simulink model "model_13"  (R2022b)
settings: Solver=VariableStepAuto  StartTime=0.0  StopTime=2000  FixedStep=1e-3  RelTol=1e-3  EnableMultiTasking=on
StopFcn:
  | ee_addSimlogTimeStamp(bdroot)
libraries: fl_lib x74, nesl_utility x53, ee_lib x22, spsRMSLib x22, eePowerMeasurement x11
(part 1 of 2)
CloseFcn:
  | try,close(h1_ee_voltreg_linear_feedback),end
  | clear h1_ee_voltreg_linear_feedback
  | try,close(h2_ee_voltreg_linear_feedback),end
  | 
  | clear simlog_ee_voltreg_linear_feedback
  | clear logsout_ee_voltreg_linear_feedback
  | clear tout
Description:
  | Linear Voltage Regulator with Feedback
settings Model: Creator=The MathWorks, Inc.  LastModifiedBy=aykut
settings SolverCC: ZeroCrossAlgorithm=Adaptive  AlgebraicLoopSolver=TrustRegion
settings DataIOCC: MaxDataPoints=15000  SaveFormat=Array  ReturnWorkspaceOutputs=off  SignalLoggingName=logsout_ee_voltreg_linear_feedback
settings OptimizationCC: ExpressionDepthLimit=2147483647  InitFltsAndDblsToZero=on  LifeSpan=inf
settings DebuggingCC: SaveWithParameterizedLinksMsg=none  UnderspecifiedInitializationDetection=Classic  MergeDetectMultiDrivingBlocksExec=none  IgnoredZcDiagnostic=none  FcnCallInpInsideContextMsg=warning  UnconnectedInputMsg=warning  UnconnectedOutputMsg=warning  UnconnectedLineMsg=warning  StateNameClashWarn=warning  SFUnexpectedBacktrackingDiag=warning  SFNoUnconditionalDefaultTransitionDiag=warning  SFExecutionAtInitializationDiag=none  SFMachineParentedDataDiag=warning  ArithmeticOperatorsInVariantConditions=warning
settings HardwareCC: ProdBitPerPointer=32  ProdBitPerSizeT=32  ProdBitPerPtrDiffT=32  ProdLargestAtomicFloat=None  ProdIntDivRoundTo=Undefined  ProdEndianess=Unspecified  ProdWordSize=32  ProdHWDeviceType=32-bit Generic
settings ModelReferenceCC: EnableRefExpFcnMdlSchedulingChecks=on  PropagateSignalLabelsOutOfModel=off
settings SFSimCC: SimUseLocalCustomCode=off  CustomCodeUndefinedFunction=UseInterfaceOnly
settings RTWCC: RTWUseLocalCustomCode=off  DLArmComputeVersion=19.05
settings CodeAppCC: StateflowObjectComments=on
settings GRTTargetCC: TargetFcnLib=ansi_tfl_tmw.mat  TargetLangStandard=C89/C90 (ANSI)  CombineOutputUpdateFcns=off  GRTInterface=on
settings ConfigComp: CovMetricSettings=dw  CovSaveCumulativeToWorkspaceVar=on  CovSaveSingleToWorkspaceVar=on  CovExternalEMLEnable=off  CovSFcnEnable=off
settings SimscapeCC: SimscapeLogType=all  SimscapeLogSimulationStatistics=on  SimscapeLogName=simlog_ee_voltreg_linear_feedback  SimscapeLogDataHistory=15000

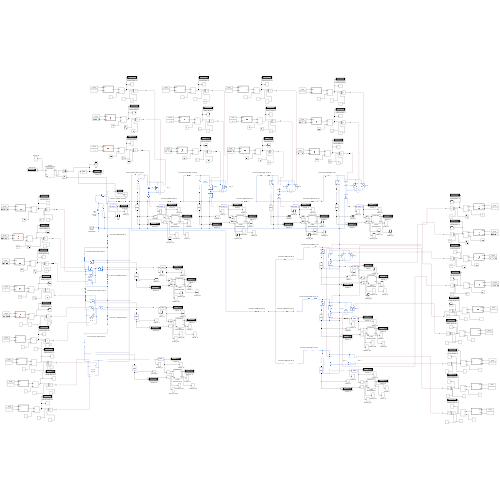
[thumbnail: Simulink's stored preview of the top-level diagram]
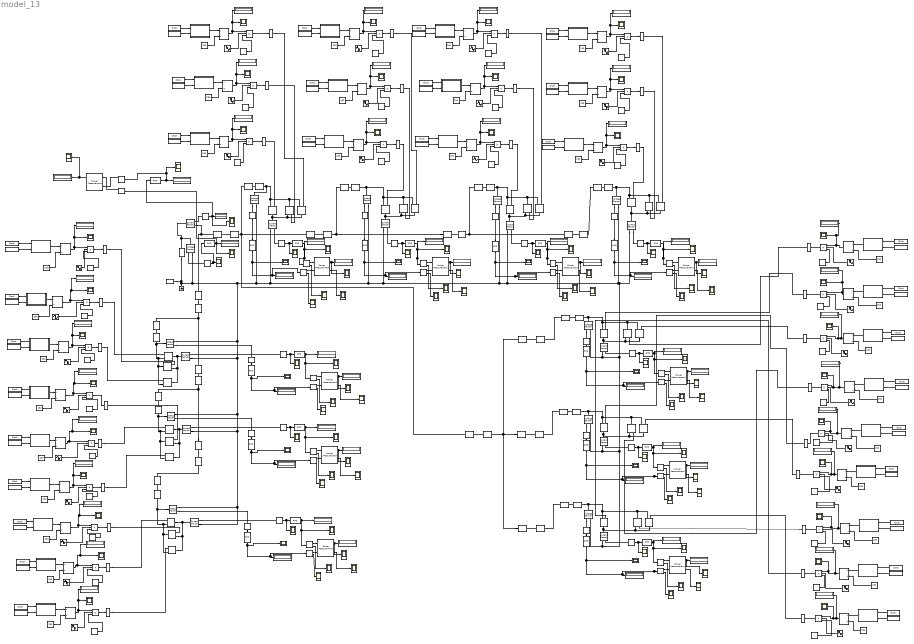
== system model_13 ==
  -Line Pair 10 (AMKA 35 52 m) : fl_lib/Electrical/Electrical Elements/Resistor  R=0.045136 Ohm  i_specify=off  i_priority=High  i=0 A  i_nominal_specify=off  i_nominal_unit=A  i_nominal_value=1  v_specify=off  v_priority=High  v=0 V  v_nominal_specify=off  v_nominal_unit=V  v_nominal_value=1
  -Line Pair 11 (AMKA 25 58 m) : fl_lib/Electrical/Electrical Elements/Resistor  R=0.0696 Ohm  i_specify=off  i_priority=High  i=0 A  i_nominal_specify=off  i_nominal_unit=A  i_nominal_value=1  v_specify=off  v_priority=High  v=0 V  v_nominal_specify=off  v_nominal_unit=V  v_nominal_value=1
  -Line Pair 9 (AMKA 35 85 m) : fl_lib/Electrical/Electrical Elements/Resistor  R=0.07378 Ohm  i_specify=off  i_priority=High  i=0 A  i_nominal_specify=off  i_nominal_unit=A  i_nominal_value=1  v_specify=off  v_priority=High  v=0 V  v_nominal_specify=off  v_nominal_unit=V  v_nominal_value=1
  -Line Pair House 2(MC 10 48 m) : fl_lib/Electrical/Electrical Elements/Resistor  R=0.08784 Ohm  i_specify=off  i_priority=High  i=0 A  i_nominal_specify=off  i_nominal_unit=A  i_nominal_value=1  v_specify=off  v_priority=High  v=0 V  v_nominal_specify=off  v_nominal_unit=V  v_nominal_value=1
  -Line Pair House 3(MC 10 34 m) : fl_lib/Electrical/Electrical Elements/Resistor  R=0.06222 Ohm  i_specify=off  i_priority=High  i=0 A  i_nominal_specify=off  i_nominal_unit=A  i_nominal_value=1  v_specify=off  v_priority=High  v=0 V  v_nominal_specify=off  v_nominal_unit=V  v_nominal_value=1
  -Line Pair House 4(MC6  4 m) : fl_lib/Electrical/Electrical Elements/Resistor  R=0.01232 Ohm  i_specify=off  i_priority=High  i=0 A  i_nominal_specify=off  i_nominal_unit=A  i_nominal_value=1  v_specify=off  v_priority=High  v=0 V  v_nominal_specify=off  v_nominal_unit=V  v_nominal_value=1
  -Line Pair House 5(MC 6 11 m) : fl_lib/Electrical/Electrical Elements/Resistor  R=0.03388 Ohm  i_specify=off  i_priority=High  i=0 A  i_nominal_specify=off  i_nominal_unit=A  i_nominal_value=1  v_specify=off  v_priority=High  v=0 V  v_nominal_specify=off  v_nominal_unit=V  v_nominal_value=1
  -Line Pair House 6(MC 10 12 m) : fl_lib/Electrical/Electrical Elements/Resistor  R=0.02196 Ohm  i_specify=off  i_priority=High  i=0 A  i_nominal_specify=off  i_nominal_unit=A  i_nominal_value=1  v_specify=off  v_priority=High  v=0 V  v_nominal_specify=off  v_nominal_unit=V  v_nominal_value=1
  Complex to Real-Imag{1..22} (22 alike) : ComplexToRealImag
  Constant{1..30} (30 alike) : Constant  Value=230
  Constant{31..60} (30 alike) : Constant  Value=sqrt(2)
  Controlled Current Source{,1..9} (10 alike) : fl_lib/Electrical/Electrical Sources/Controlled Current Source
  Current Sensor{,1..10} (11 alike) : fl_lib/Electrical/Electrical Sensors/Current Sensor
  Digital Clock{1..30} (30 alike) : DigitalClock
  Divide{1..30} (30 alike) : Product  Inputs=*/
  ERef : fl_lib/Electrical/Electrical Elements/Electrical Reference
  EV_{1..10} (10 alike) : fl_lib/Electrical/Electrical Sources/Controlled Current Source
  From Workspace : FromWorkspace  VariableName=house1_load_array  OutDataTypeStr=double  Interpolate=off  OutputAfterFinalValue=Holding final value
  From Workspace1 : FromWorkspace  VariableName=house1_pv_array  OutDataTypeStr=double  Interpolate=off  OutputAfterFinalValue=Holding final value
  From Workspace10 : FromWorkspace  VariableName=house9_load_array  OutDataTypeStr=double  Interpolate=off  OutputAfterFinalValue=Holding final value
  From Workspace11 : FromWorkspace  VariableName=house9_pv_array  OutDataTypeStr=double  Interpolate=off  OutputAfterFinalValue=Holding final value
  From Workspace12 : FromWorkspace  VariableName=house10_load_array  OutDataTypeStr=double  Interpolate=off  OutputAfterFinalValue=Holding final value
  From Workspace13 : FromWorkspace  VariableName=house10_pv_array  OutDataTypeStr=double  Interpolate=off  OutputAfterFinalValue=Holding final value
  From Workspace14 : FromWorkspace  VariableName=house5_load_array  OutDataTypeStr=double  Interpolate=off  OutputAfterFinalValue=Holding final value
  From Workspace15 : FromWorkspace  VariableName=house5_pv_array  OutDataTypeStr=double  Interpolate=off  OutputAfterFinalValue=Holding final value
  From Workspace16 : FromWorkspace  VariableName=house6_load_array  OutDataTypeStr=double  Interpolate=off  OutputAfterFinalValue=Holding final value
  From Workspace17 : FromWorkspace  VariableName=house6_pv_array  OutDataTypeStr=double  Interpolate=off  OutputAfterFinalValue=Holding final value
  From Workspace18 : FromWorkspace  VariableName=house7_load_array  OutDataTypeStr=double  Interpolate=off  OutputAfterFinalValue=Holding final value
  From Workspace19 : FromWorkspace  VariableName=house7_pv_array  OutDataTypeStr=double  Interpolate=off  OutputAfterFinalValue=Holding final value
  From Workspace2 : FromWorkspace  VariableName=house2_load_array  OutDataTypeStr=double  Interpolate=off  OutputAfterFinalValue=Holding final value
  From Workspace20 : FromWorkspace  VariableName=house1_ev_array  OutDataTypeStr=double  Interpolate=off  OutputAfterFinalValue=Holding final value
  From Workspace21 : FromWorkspace  VariableName=house2_ev_array  OutDataTypeStr=double  Interpolate=off  OutputAfterFinalValue=Holding final value
  From Workspace22 : FromWorkspace  VariableName=house3_ev_array  OutDataTypeStr=double  Interpolate=off  OutputAfterFinalValue=Holding final value
  From Workspace23 : FromWorkspace  VariableName=house4_ev_array  OutDataTypeStr=double  Interpolate=off  OutputAfterFinalValue=Holding final value
  From Workspace24 : FromWorkspace  VariableName=house5_ev_array  OutDataTypeStr=double  Interpolate=off  OutputAfterFinalValue=Holding final value
  From Workspace25 : FromWorkspace  VariableName=house6_ev_array  OutDataTypeStr=double  Interpolate=off  OutputAfterFinalValue=Holding final value
  From Workspace26 : FromWorkspace  VariableName=house7_ev_array  OutDataTypeStr=double  Interpolate=off  OutputAfterFinalValue=Holding final value
  From Workspace27 : FromWorkspace  VariableName=house8_ev_array  OutDataTypeStr=double  Interpolate=off  OutputAfterFinalValue=Holding final value
  From Workspace28 : FromWorkspace  VariableName=house9_ev_array  OutDataTypeStr=double  Interpolate=off  OutputAfterFinalValue=Holding final value
  From Workspace29 : FromWorkspace  VariableName=house10_ev_array  OutDataTypeStr=double  Interpolate=off  OutputAfterFinalValue=Holding final value
  From Workspace3 : FromWorkspace  VariableName=house2_pv_array  OutDataTypeStr=double  Interpolate=off  OutputAfterFinalValue=Holding final value
  From Workspace4 : FromWorkspace  VariableName=house3_load_array  OutDataTypeStr=double  Interpolate=off  OutputAfterFinalValue=Holding final value
  From Workspace5 : FromWorkspace  VariableName=house3_pv_array  OutDataTypeStr=double  Interpolate=off  OutputAfterFinalValue=Holding final value
  From Workspace6 : FromWorkspace  VariableName=house4_load_array  OutDataTypeStr=double  Interpolate=off  OutputAfterFinalValue=Holding final value
  From Workspace7 : FromWorkspace  VariableName=house4_pv_array  OutDataTypeStr=double  Interpolate=off  OutputAfterFinalValue=Holding final value
  From Workspace8 : FromWorkspace  VariableName=house8_load_array  OutDataTypeStr=double  Interpolate=off  OutputAfterFinalValue=Holding final value
  From Workspace9 : FromWorkspace  VariableName=house8_pv_array  OutDataTypeStr=double  Interpolate=off  OutputAfterFinalValue=Holding final value
  Ih10rms_d : Display
  Ih10rms_s1 : Scope
  Ih10rms_s2 : Scope
  Ih1rms_d{,1..3} (4 alike) : Display
  Ih1rms_s1 : Scope
  Ih1rms_s2 : Scope
  Ih1rms_s3 : Scope
  Ih2rms_d : Display
  Ih2rms_s1 : Scope
  Ih2rms_s2 : Scope
  Ih3rms_d : Display
  Ih3rms_s1 : Scope
  Ih3rms_s2 : Scope
  Ih4rms_d : Display
  Ih4rms_s1 : Scope
  Ih4rms_s2 : Scope
  Ih5rms_d : Display
  Ih5rms_s1 : Scope
  Ih5rms_s2 : Scope
  Ih6rms_d : Display
  Ih6rms_s1 : Scope
  Ih6rms_s2 : Scope
  Ih7rms_d : Display
  Ih7rms_s1 : Scope
  Ih7rms_s2 : Scope
  Ih8rms_d : Display
  Ih8rms_s1 : Scope
  Ih8rms_s2 : Scope
  Ih9rms_d : Display
  Ih9rms_s1 : Scope
  Ih9rms_s2 : Scope
  Inductor : ee_lib/Passive/Inductor  l=2.947770700636943e-5 H  enable_L_tol=0  L_tol=20  tol_distribution=1  nSigma=4  r=0 Ohm  g=0 1/Ohm  enable_operating_limits=0  operating_limit_action=2  max_working_current=1 A  power_rating=1 W  enable_faults=0  fault_action=1  lambdaPercent=50  k_faulted=0.9999  turnsShort=0  openCct=0  groundShort=0  groundShortG=0 1/Ohm  tau_fault=1e-3 s  enable_temporal_fault=0  t_fault=1 s  enable_behavioral_fault=0  max_permissible_voltage=100 V  n_fail_on_voltage=1  max_permissible_current=1 A  t_fail_on_current=1 s  i_L_specify=off  i_L_priority=High  i_L=0 A  i_L_nominal_specify=off  i_L_nominal_unit=A  i_L_nominal_value=1
  Inductor1 : ee_lib/Passive/Inductor  l=1.064968152866242e-5 H  enable_L_tol=0  L_tol=20  tol_distribution=1  nSigma=4  r=0 Ohm  g=0 1/Ohm  enable_operating_limits=0  operating_limit_action=2  max_working_current=1 A  power_rating=1 W  enable_faults=0  fault_action=1  lambdaPercent=50  k_faulted=0.9999  turnsShort=0  openCct=0  groundShort=0  groundShortG=0 1/Ohm  tau_fault=1e-3 s  enable_temporal_fault=0  t_fault=1 s  enable_behavioral_fault=0  max_permissible_voltage=100 V  n_fail_on_voltage=1  max_permissible_current=1 A  t_fail_on_current=1 s  i_L_specify=off  i_L_priority=High  i_L=0 A  i_L_nominal_specify=off  i_L_nominal_unit=A  i_L_nominal_value=1
  Inductor10 : ee_lib/Passive/Inductor  l=1.547770700636943e-5 H  enable_L_tol=0  L_tol=20  tol_distribution=1  nSigma=4  r=0 Ohm  g=0 1/Ohm  enable_operating_limits=0  operating_limit_action=2  max_working_current=1 A  power_rating=1 W  enable_faults=0  fault_action=1  lambdaPercent=50  k_faulted=0.9999  turnsShort=0  openCct=0  groundShort=0  groundShortG=0 1/Ohm  tau_fault=1e-3 s  enable_temporal_fault=0  t_fault=1 s  enable_behavioral_fault=0  max_permissible_voltage=100 V  n_fail_on_voltage=1  max_permissible_current=1 A  t_fail_on_current=1 s  i_L_specify=off  i_L_priority=High  i_L=0 A  i_L_nominal_specify=off  i_L_nominal_unit=A  i_L_nominal_value=1
  Inductor11 : ee_lib/Passive/Inductor  l=4.537579617834395e-5 H  enable_L_tol=0  L_tol=20  tol_distribution=1  nSigma=4  r=0 Ohm  g=0 1/Ohm  enable_operating_limits=0  operating_limit_action=2  max_working_current=1 A  power_rating=1 W  enable_faults=0  fault_action=1  lambdaPercent=50  k_faulted=0.9999  turnsShort=0  openCct=0  groundShort=0  groundShortG=0 1/Ohm  tau_fault=1e-3 s  enable_temporal_fault=0  t_fault=1 s  enable_behavioral_fault=0  max_permissible_voltage=100 V  n_fail_on_voltage=1  max_permissible_current=1 A  t_fail_on_current=1 s  i_L_specify=off  i_L_priority=High  i_L=0 A  i_L_nominal_specify=off  i_L_nominal_unit=A  i_L_nominal_value=1
  Inductor12 : ee_lib/Passive/Inductor  l=1.092993630573248e-5 H  enable_L_tol=0  L_tol=20  tol_distribution=1  nSigma=4  r=0 Ohm  g=0 1/Ohm  enable_operating_limits=0  operating_limit_action=2  max_working_current=1 A  power_rating=1 W  enable_faults=0  fault_action=1  lambdaPercent=50  k_faulted=0.9999  turnsShort=0  openCct=0  groundShort=0  groundShortG=0 1/Ohm  tau_fault=1e-3 s  enable_temporal_fault=0  t_fault=1 s  enable_behavioral_fault=0  max_permissible_voltage=100 V  n_fail_on_voltage=1  max_permissible_current=1 A  t_fail_on_current=1 s  i_L_specify=off  i_L_priority=High  i_L=0 A  i_L_nominal_specify=off  i_L_nominal_unit=A  i_L_nominal_value=1
  Inductor13 : ee_lib/Passive/Inductor  l=3.152866242038217e-6 H  enable_L_tol=0  L_tol=20  tol_distribution=1  nSigma=4  r=0 Ohm  g=0 1/Ohm  enable_operating_limits=0  operating_limit_action=2  max_working_current=1 A  power_rating=1 W  enable_faults=0  fault_action=1  lambdaPercent=50  k_faulted=0.9999  turnsShort=0  openCct=0  groundShort=0  groundShortG=0 1/Ohm  tau_fault=1e-3 s  enable_temporal_fault=0  t_fault=1 s  enable_behavioral_fault=0  max_permissible_voltage=100 V  n_fail_on_voltage=1  max_permissible_current=1 A  t_fail_on_current=1 s  i_L_specify=off  i_L_priority=High  i_L=0 A  i_L_nominal_specify=off  i_L_nominal_unit=A  i_L_nominal_value=1
  Inductor14 : ee_lib/Passive/Inductor  l=3.363057324840764e-6 H  enable_L_tol=0  L_tol=20  tol_distribution=1  nSigma=4  r=0 Ohm  g=0 1/Ohm  enable_operating_limits=0  operating_limit_action=2  max_working_current=1 A  power_rating=1 W  enable_faults=0  fault_action=1  lambdaPercent=50  k_faulted=0.9999  turnsShort=0  openCct=0  groundShort=0  groundShortG=0 1/Ohm  tau_fault=1e-3 s  enable_temporal_fault=0  t_fault=1 s  enable_behavioral_fault=0  max_permissible_voltage=100 V  n_fail_on_voltage=1  max_permissible_current=1 A  t_fail_on_current=1 s  i_L_specify=off  i_L_priority=High  i_L=0 A  i_L_nominal_specify=off  i_L_nominal_unit=A  i_L_nominal_value=1
  Inductor15 : ee_lib/Passive/Inductor  l=1.064968152866242e-5 H  enable_L_tol=0  L_tol=20  tol_distribution=1  nSigma=4  r=0 Ohm  g=0 1/Ohm  enable_operating_limits=0  operating_limit_action=2  max_working_current=1 A  power_rating=1 W  enable_faults=0  fault_action=1  lambdaPercent=50  k_faulted=0.9999  turnsShort=0  openCct=0  groundShort=0  groundShortG=0 1/Ohm  tau_fault=1e-3 s  enable_temporal_fault=0  t_fault=1 s  enable_behavioral_fault=0  max_permissible_voltage=100 V  n_fail_on_voltage=1  max_permissible_current=1 A  t_fail_on_current=1 s  i_L_specify=off  i_L_priority=High  i_L=0 A  i_L_nominal_specify=off  i_L_nominal_unit=A  i_L_nominal_value=1
  Inductor16 : ee_lib/Passive/Inductor  l=8.127388535031847e-6 H  enable_L_tol=0  L_tol=20  tol_distribution=1  nSigma=4  r=0 Ohm  g=0 1/Ohm  enable_operating_limits=0  operating_limit_action=2  max_working_current=1 A  power_rating=1 W  enable_faults=0  fault_action=1  lambdaPercent=50  k_faulted=0.9999  turnsShort=0  openCct=0  groundShort=0  groundShortG=0 1/Ohm  tau_fault=1e-3 s  enable_temporal_fault=0  t_fault=1 s  enable_behavioral_fault=0  max_permissible_voltage=100 V  n_fail_on_voltage=1  max_permissible_current=1 A  t_fail_on_current=1 s  i_L_specify=off  i_L_priority=High  i_L=0 A  i_L_nominal_specify=off  i_L_nominal_unit=A  i_L_nominal_value=1
  Inductor17 : ee_lib/Passive/Inductor  l=1.722292993630573e-5 H  enable_L_tol=0  L_tol=20  tol_distribution=1  nSigma=4  r=0 Ohm  g=0 1/Ohm  enable_operating_limits=0  operating_limit_action=2  max_working_current=1 A  power_rating=1 W  enable_faults=0  fault_action=1  lambdaPercent=50  k_faulted=0.9999  turnsShort=0  openCct=0  groundShort=0  groundShortG=0 1/Ohm  tau_fault=1e-3 s  enable_temporal_fault=0  t_fault=1 s  enable_behavioral_fault=0  max_permissible_voltage=100 V  n_fail_on_voltage=1  max_permissible_current=1 A  t_fail_on_current=1 s  i_L_specify=off  i_L_priority=High  i_L=0 A  i_L_nominal_specify=off  i_L_nominal_unit=A  i_L_nominal_value=1
  Inductor18 : ee_lib/Passive/Inductor  l=9.808917197452229e-6 H  enable_L_tol=0  L_tol=20  tol_distribution=1  nSigma=4  r=0 Ohm  g=0 1/Ohm  enable_operating_limits=0  operating_limit_action=2  max_working_current=1 A  power_rating=1 W  enable_faults=0  fault_action=1  lambdaPercent=50  k_faulted=0.9999  turnsShort=0  openCct=0  groundShort=0  groundShortG=0 1/Ohm  tau_fault=1e-3 s  enable_temporal_fault=0  t_fault=1 s  enable_behavioral_fault=0  max_permissible_voltage=100 V  n_fail_on_voltage=1  max_permissible_current=1 A  t_fail_on_current=1 s  i_L_specify=off  i_L_priority=High  i_L=0 A  i_L_nominal_specify=off  i_L_nominal_unit=A  i_L_nominal_value=1
  Inductor19 : ee_lib/Passive/Inductor  l=1.95796178343949e-5 H  enable_L_tol=0  L_tol=20  tol_distribution=1  nSigma=4  r=0 Ohm  g=0 1/Ohm  enable_operating_limits=0  operating_limit_action=2  max_working_current=1 A  power_rating=1 W  enable_faults=0  fault_action=1  lambdaPercent=50  k_faulted=0.9999  turnsShort=0  openCct=0  groundShort=0  groundShortG=0 1/Ohm  tau_fault=1e-3 s  enable_temporal_fault=0  t_fault=1 s  enable_behavioral_fault=0  max_permissible_voltage=100 V  n_fail_on_voltage=1  max_permissible_current=1 A  t_fail_on_current=1 s  i_L_specify=off  i_L_priority=High  i_L=0 A  i_L_nominal_specify=off  i_L_nominal_unit=A  i_L_nominal_value=1
  Inductor2 : ee_lib/Passive/Inductor  l=1.987261146496815e-5 H  enable_L_tol=0  L_tol=20  tol_distribution=1  nSigma=4  r=0 Ohm  g=0 1/Ohm  enable_operating_limits=0  operating_limit_action=2  max_working_current=1 A  power_rating=1 W  enable_faults=0  fault_action=1  lambdaPercent=50  k_faulted=0.9999  turnsShort=0  openCct=0  groundShort=0  groundShortG=0 1/Ohm  tau_fault=1e-3 s  enable_temporal_fault=0  t_fault=1 s  enable_behavioral_fault=0  max_permissible_voltage=100 V  n_fail_on_voltage=1  max_permissible_current=1 A  t_fail_on_current=1 s  i_L_specify=off  i_L_priority=High  i_L=0 A  i_L_nominal_specify=off  i_L_nominal_unit=A  i_L_nominal_value=1
  Inductor20 : ee_lib/Passive/Inductor  l=1.146496815286624e-5 H  enable_L_tol=0  L_tol=20  tol_distribution=1  nSigma=4  r=0 Ohm  g=0 1/Ohm  enable_operating_limits=0  operating_limit_action=2  max_working_current=1 A  power_rating=1 W  enable_faults=0  fault_action=1  lambdaPercent=50  k_faulted=0.9999  turnsShort=0  openCct=0  groundShort=0  groundShortG=0 1/Ohm  tau_fault=1e-3 s  enable_temporal_fault=0  t_fault=1 s  enable_behavioral_fault=0  max_permissible_voltage=100 V  n_fail_on_voltage=1  max_permissible_current=1 A  t_fail_on_current=1 s  i_L_specify=off  i_L_priority=High  i_L=0 A  i_L_nominal_specify=off  i_L_nominal_unit=A  i_L_nominal_value=1
  Inductor3 : ee_lib/Passive/Inductor  l=3.146496815286624e-5 H  enable_L_tol=0  L_tol=20  tol_distribution=1  nSigma=4  r=0 Ohm  g=0 1/Ohm  enable_operating_limits=0  operating_limit_action=2  max_working_current=1 A  power_rating=1 W  enable_faults=0  fault_action=1  lambdaPercent=50  k_faulted=0.9999  turnsShort=0  openCct=0  groundShort=0  groundShortG=0 1/Ohm  tau_fault=1e-3 s  enable_temporal_fault=0  t_fault=1 s  enable_behavioral_fault=0  max_permissible_voltage=100 V  n_fail_on_voltage=1  max_permissible_current=1 A  t_fail_on_current=1 s  i_L_specify=off  i_L_priority=High  i_L=0 A  i_L_nominal_specify=off  i_L_nominal_unit=A  i_L_nominal_value=1
  Inductor4 : ee_lib/Passive/Inductor  l=1.600254777070064e-4 H  enable_L_tol=0  L_tol=20  tol_distribution=1  nSigma=4  r=0 Ohm  g=0 1/Ohm  enable_operating_limits=0  operating_limit_action=2  max_working_current=1 A  power_rating=1 W  enable_faults=0  fault_action=1  lambdaPercent=50  k_faulted=0.9999  turnsShort=0  openCct=0  groundShort=0  groundShortG=0 1/Ohm  tau_fault=1e-3 s  enable_temporal_fault=0  t_fault=1 s  enable_behavioral_fault=0  max_permissible_voltage=100 V  n_fail_on_voltage=1  max_permissible_current=1 A  t_fail_on_current=1 s  i_L_specify=off  i_L_priority=High  i_L=0 A  i_L_nominal_specify=off  i_L_nominal_unit=A  i_L_nominal_value=1
  Inductor5 : ee_lib/Passive/Inductor  l=1.345222929936306e-5 H  enable_L_tol=0  L_tol=20  tol_distribution=1  nSigma=4  r=0 Ohm  g=0 1/Ohm  enable_operating_limits=0  operating_limit_action=2  max_working_current=1 A  power_rating=1 W  enable_faults=0  fault_action=1  lambdaPercent=50  k_faulted=0.9999  turnsShort=0  openCct=0  groundShort=0  groundShortG=0 1/Ohm  tau_fault=1e-3 s  enable_temporal_fault=0  t_fault=1 s  enable_behavioral_fault=0  max_permissible_voltage=100 V  n_fail_on_voltage=1  max_permissible_current=1 A  t_fail_on_current=1 s  i_L_specify=off  i_L_priority=High  i_L=0 A  i_L_nominal_specify=off  i_L_nominal_unit=A  i_L_nominal_value=1
  Inductor6 : ee_lib/Passive/Inductor  l=9.528662420382166e-6 H  enable_L_tol=0  L_tol=20  tol_distribution=1  nSigma=4  r=0 Ohm  g=0 1/Ohm  enable_operating_limits=0  operating_limit_action=2  max_working_current=1 A  power_rating=1 W  enable_faults=0  fault_action=1  lambdaPercent=50  k_faulted=0.9999  turnsShort=0  openCct=0  groundShort=0  groundShortG=0 1/Ohm  tau_fault=1e-3 s  enable_temporal_fault=0  t_fault=1 s  enable_behavioral_fault=0  max_permissible_voltage=100 V  n_fail_on_voltage=1  max_permissible_current=1 A  t_fail_on_current=1 s  i_L_specify=off  i_L_priority=High  i_L=0 A  i_L_nominal_specify=off  i_L_nominal_unit=A  i_L_nominal_value=1
  Inductor7 : ee_lib/Passive/Inductor  l=1.146496815286624e-6 H  enable_L_tol=0  L_tol=20  tol_distribution=1  nSigma=4  r=0 Ohm  g=0 1/Ohm  enable_operating_limits=0  operating_limit_action=2  max_working_current=1 A  power_rating=1 W  enable_faults=0  fault_action=1  lambdaPercent=50  k_faulted=0.9999  turnsShort=0  openCct=0  groundShort=0  groundShortG=0 1/Ohm  tau_fault=1e-3 s  enable_temporal_fault=0  t_fault=1 s  enable_behavioral_fault=0  max_permissible_voltage=100 V  n_fail_on_voltage=1  max_permissible_current=1 A  t_fail_on_current=1 s  i_L_specify=off  i_L_priority=High  i_L=0 A  i_L_nominal_specify=off  i_L_nominal_unit=A  i_L_nominal_value=1
  Inductor8 : ee_lib/Passive/Inductor  l=0.0000273407643312 H  enable_L_tol=0  L_tol=20  tol_distribution=1  nSigma=4  r=0 Ohm  g=0 1/Ohm  enable_operating_limits=0  operating_limit_action=2  max_working_current=1 A  power_rating=1 W  enable_faults=0  fault_action=1  lambdaPercent=50  k_faulted=0.9999  turnsShort=0  openCct=0  groundShort=0  groundShortG=0 1/Ohm  tau_fault=1e-3 s  enable_temporal_fault=0  t_fault=1 s  enable_behavioral_fault=0  max_permissible_voltage=100 V  n_fail_on_voltage=1  max_permissible_current=1 A  t_fail_on_current=1 s  i_L_specify=off  i_L_priority=High  i_L=0 A  i_L_nominal_specify=off  i_L_nominal_unit=A  i_L_nominal_value=1
  Inductor9 : ee_lib/Passive/Inductor  l=8.214012738853503e-5 H  enable_L_tol=0  L_tol=20  tol_distribution=1  nSigma=4  r=0 Ohm  g=0 1/Ohm  enable_operating_limits=0  operating_limit_action=2  max_working_current=1 A  power_rating=1 W  enable_faults=0  fault_action=1  lambdaPercent=50  k_faulted=0.9999  turnsShort=0  openCct=0  groundShort=0  groundShortG=0 1/Ohm  tau_fault=1e-3 s  enable_temporal_fault=0  t_fault=1 s  enable_behavioral_fault=0  max_permissible_voltage=100 V  n_fail_on_voltage=1  max_permissible_current=1 A  t_fail_on_current=1 s  i_L_specify=off  i_L_priority=High  i_L=0 A  i_L_nominal_specify=off  i_L_nominal_unit=A  i_L_nominal_value=1
  Itr : Scope
  Itr1 : Scope
  Line Pair 1 (AMKA 35 89 m) : fl_lib/Electrical/Electrical Elements/Resistor  R=0.077252 Ohm  i_specify=off  i_priority=High  i=0 A  i_nominal_specify=off  i_nominal_unit=A  i_nominal_value=1  v_specify=off  v_priority=High  v=0 V  v_nominal_specify=off  v_nominal_unit=V  v_nominal_value=1
  Line Pair 2 (AMKA 35 60 m) : fl_lib/Electrical/Electrical Elements/Resistor  R=0.05208 Ohm  i_specify=off  i_priority=High  i=0 A  i_nominal_specify=off  i_nominal_unit=A  i_nominal_value=1  v_specify=off  v_priority=High  v=0 V  v_nominal_specify=off  v_nominal_unit=V  v_nominal_value=1
  Line Pair 3 (AMKA 35 95 m) : fl_lib/Electrical/Electrical Elements/Resistor  R=0.08246 Ohm  i_specify=off  i_priority=High  i=0 A  i_nominal_specify=off  i_nominal_unit=A  i_nominal_value=1  v_specify=off  v_priority=High  v=0 V  v_nominal_specify=off  v_nominal_unit=V  v_nominal_value=1
  Line Pair 4 (AXMK 50 571 m) : fl_lib/Electrical/Electrical Elements/Resistor  R=0.366011 Ohm  i_specify=off  i_priority=High  i=0 A  i_nominal_specify=off  i_nominal_unit=A  i_nominal_value=1  v_specify=off  v_priority=High  v=0 V  v_nominal_specify=off  v_nominal_unit=V  v_nominal_value=1
  Line Pair 5 (AMKA 35 248 m) : fl_lib/Electrical/Electrical Elements/Resistor  R=0.215264 Ohm  i_specify=off  i_priority=High  i=0 A  i_nominal_specify=off  i_nominal_unit=A  i_nominal_value=1  v_specify=off  v_priority=High  v=0 V  v_nominal_specify=off  v_nominal_unit=V  v_nominal_value=1
  Line Pair 6 (AMKA 16 45 m) : fl_lib/Electrical/Electrical Elements/Resistor  R=0.08595 Ohm  i_specify=off  i_priority=High  i=0 A  i_nominal_specify=off  i_nominal_unit=A  i_nominal_value=1  v_specify=off  v_priority=High  v=0 V  v_nominal_specify=off  v_nominal_unit=V  v_nominal_value=1
  Line Pair 7 (AMKA 35 137 m) : fl_lib/Electrical/Electrical Elements/Resistor  R=0.118916 Ohm  i_specify=off  i_priority=High  i=0 A  i_nominal_specify=off  i_nominal_unit=A  i_nominal_value=1  v_specify=off  v_priority=High  v=0 V  v_nominal_specify=off  v_nominal_unit=V  v_nominal_value=1
  Line Pair 8 (AMKA 35 33 m) : fl_lib/Electrical/Electrical Elements/Resistor  R=0.028644 Ohm  i_specify=off  i_priority=High  i=0 A  i_nominal_specify=off  i_nominal_unit=A  i_nominal_value=1  v_specify=off  v_priority=High  v=0 V  v_nominal_specify=off  v_nominal_unit=V  v_nominal_value=1
  Line Pair House 1 (MC 10 38 m) : fl_lib/Electrical/Electrical Elements/Resistor  R=0.06954 Ohm  i_specify=off  i_priority=High  i=0 A  i_nominal_specify=off  i_nominal_unit=A  i_nominal_value=1  v_specify=off  v_priority=High  v=0 V  v_nominal_specify=off  v_nominal_unit=V  v_nominal_value=1
  Line Pair House 10 (MC 6 40 m) : fl_lib/Electrical/Electrical Elements/Resistor  R=0.1232 Ohm  i_specify=off  i_priority=High  i=0 A  i_nominal_specify=off  i_nominal_unit=A  i_nominal_value=1  v_specify=off  v_priority=High  v=0 V  v_nominal_specify=off  v_nominal_unit=V  v_nominal_value=1
  Line Pair House 7(MC 10 38 m) : fl_lib/Electrical/Electrical Elements/Resistor  R=0.06954 Ohm  i_specify=off  i_priority=High  i=0 A  i_nominal_specify=off  i_nominal_unit=A  i_nominal_value=1  v_specify=off  v_priority=High  v=0 V  v_nominal_specify=off  v_nominal_unit=V  v_nominal_value=1
  Line Pair House 8 (MC 10 29 m) : fl_lib/Electrical/Electrical Elements/Resistor  R=0.05307 Ohm  i_specify=off  i_priority=High  i=0 A  i_nominal_specify=off  i_nominal_unit=A  i_nominal_value=1  v_specify=off  v_priority=High  v=0 V  v_nominal_specify=off  v_nominal_unit=V  v_nominal_value=1
  Line Pair House 9 (MC 10 35 m) : fl_lib/Electrical/Electrical Elements/Resistor  R=0.06405 Ohm  i_specify=off  i_priority=High  i=0 A  i_nominal_specify=off  i_nominal_unit=A  i_nominal_value=1  v_specify=off  v_priority=High  v=0 V  v_nominal_specify=off  v_nominal_unit=V  v_nominal_value=1
  MATLAB Function1 : MATLAB Function  TreatAsAtomicUnit=on
  MATLAB Function10 : MATLAB Function  TreatAsAtomicUnit=on
  MATLAB Function11 : MATLAB Function  TreatAsAtomicUnit=on
  MATLAB Function12 : MATLAB Function  TreatAsAtomicUnit=on
  MATLAB Function13 : MATLAB Function  TreatAsAtomicUnit=on
  MATLAB Function14 : MATLAB Function  TreatAsAtomicUnit=on
  MATLAB Function15 : MATLAB Function  TreatAsAtomicUnit=on
  MATLAB Function16 : MATLAB Function  TreatAsAtomicUnit=on
  MATLAB Function17 : MATLAB Function  TreatAsAtomicUnit=on
  MATLAB Function18 : MATLAB Function  TreatAsAtomicUnit=on
  MATLAB Function19 : MATLAB Function  TreatAsAtomicUnit=on
  MATLAB Function2 : MATLAB Function  TreatAsAtomicUnit=on
  MATLAB Function20 : MATLAB Function  TreatAsAtomicUnit=on
  MATLAB Function21 : MATLAB Function  TreatAsAtomicUnit=on
  MATLAB Function22 : MATLAB Function  TreatAsAtomicUnit=on
  MATLAB Function23 : MATLAB Function  TreatAsAtomicUnit=on
  MATLAB Function24 : MATLAB Function  TreatAsAtomicUnit=on
  MATLAB Function25 : MATLAB Function  TreatAsAtomicUnit=on
  MATLAB Function26 : MATLAB Function  TreatAsAtomicUnit=on
  MATLAB Function27 : MATLAB Function  TreatAsAtomicUnit=on
  MATLAB Function28 : MATLAB Function  TreatAsAtomicUnit=on
  MATLAB Function29 : MATLAB Function  TreatAsAtomicUnit=on
  MATLAB Function3 : MATLAB Function  TreatAsAtomicUnit=on
  MATLAB Function30 : MATLAB Function  TreatAsAtomicUnit=on
  MATLAB Function4 : MATLAB Function  TreatAsAtomicUnit=on
  MATLAB Function5 : MATLAB Function  TreatAsAtomicUnit=on
  MATLAB Function6 : MATLAB Function  TreatAsAtomicUnit=on
  MATLAB Function7 : MATLAB Function  TreatAsAtomicUnit=on
  MATLAB Function8 : MATLAB Function  TreatAsAtomicUnit=on
  MATLAB Function9 : MATLAB Function  TreatAsAtomicUnit=on
  PV_{1..10} (10 alike) : fl_lib/Electrical/Electrical Sources/Controlled Current Source
  Ph10rms_d : Display
  Ph10rms_s : Scope
  Ph10rms_s10 : Scope
  Ph10rms_s10I : Scope
  Ph10rms_s10V : Scope
  Ph1rms_d : Display
  Ph1rms_d1 : Display
  Ph1rms_s{,1..2,7} (4 alike) : Scope
  Ph1rms_s1I : Scope
  Ph1rms_s1V : Scope
  Ph2rms_d : Display
  Ph2rms_s : Scope
  Ph2rms_s2 : Scope
  Ph2rms_s2I : Scope
  Ph2rms_s2V : Scope
  Ph3rms_d : Display
  Ph3rms_s : Scope
  Ph3rms_s3 : Scope
  Ph3rms_s3I : Scope
  Ph3rms_s3V : Scope
  Ph4rms_d : Display
  Ph4rms_s : Scope
  Ph4rms_s4 : Scope
  Ph4rms_s4I : Scope
  Ph4rms_s4V : Scope
  Ph5rms_d : Display
  Ph5rms_s : Scope
  Ph5rms_s5 : Scope
  Ph5rms_s5I : Scope
  Ph5rms_s5V : Scope
  Ph6rms_d : Display
  Ph6rms_s : Scope
  Ph6rms_s6 : Scope
  Ph6rms_s6I : Scope
  Ph6rms_s6V : Scope
  Ph7rms_d : Display
  Ph7rms_s : Scope
  Ph7rms_s7I : Scope
  Ph7rms_s7V : Scope
  Ph8rms_d : Display
  Ph8rms_s : Scope
  Ph8rms_s8 : Scope
  Ph8rms_s8I : Scope
  Ph8rms_s8V : Scope
  Ph9rms_d : Display
  Ph9rms_s : Scope
  Ph9rms_s9 : Scope
  Ph9rms_s9I : Scope
  Ph9rms_s9V : Scope
  Power Measurement{1..11} (11 alike) : eePowerMeasurement/Power Measurement  LabelModeActiveChoice=Continuous  F=50  K=[0]  Ts=0
  Product{1..30} (30 alike) : Product  Inputs=3
  RMS{1..22} (22 alike) : spsRMSLib/RMS  TrueRMS=on  Freq=50  RMSInit=0  Ts=0
  Scope{1..30} (30 alike) : Scope
  Simulink-PS Converter{,1..29} (30 alike) : nesl_utility/Simulink-PS Converter  PhysicalDomain=network_engine_domain  SubClassName=ps_input  LeftPortType=input  RightPortType=output  PseudoPeriodic=off  Frequencies=[]  NoiseDistribution=none  NoiseParameters=[]  Unit=1  AffineConversion=off  FilteringAndDerivatives=filter  SimscapeFilterOrder=1  InputFilterTimeConstant=0.001  UdotUserProvided=1
  Sine Wave{1..30} (30 alike) : Sin  SineType=Sample based  Frequency=50  SampleTime=.002
  Solver Configuration : nesl_utility/Solver Configuration  PhysicalDomain=network_engine_domain  SubClassName=solver  LeftPortType=input  RightPortType=generic  Tones=[]  Harmonics=[]  SimulateNoise=off  Profile=off  UseLocalSampling=off  EnableSwitchedLinearOptims=on  FrequencyDomain=off  UseCCode=off  RelTol=0.001  AbsTol=1e-06  MinStep=1e-09  ToWorkspace=off  RevertToSquareIcSolve=off  NumHomotopyIterations=100  PhasorMode=off  PhasorModeNumHarmonics=1  ConsistencySolver=NEWTON_FTOL  IndexReductionMethod=DerivativeReplacement  DoDC=off  ResidualTolerance=1e-9  ConsistencyTolSource=GLOBAL  ConsistencyAbsTol=0.001  ConsistencyRelTol=0.001  ConsistencyTolFactor=0.001  UseLocalSolver=on  LocalSolverChoice=NE_BACKWARD_EULER_ADVANCER  ResolveIndetEquations=on  FunctionEvalNumThread=1  LocalSolverSampleTime=.002  DoFixedCost=on  MaxNonlinIter=3  MaxModeIter=2  ComputeImpulses=off  ImpulseIterations=2  LinearAlgebra=auto  LinearAlgebraNumThread=0  EquationFormulation=NE_TIME_EF  DelaysMemoryBudget=1024  AutomaticFiltering=on  FilteringTimeConstant=0.001  PartitionStorageMethod=AS_NEEDED  PartitionMemoryBudget=1024  PartitionMethod=FAST
  VSrc : ee_lib/Sources/Voltage Source  dc_voltage=0 V  ac_voltage=324 V  ac_shift=0 deg  ac_frequency=50 Hz  noise_mode=0  PSD=0 V^2/Hz  sample_time=0.001 s  repeatability=1  user_seed=0  auto_seed=3142723716  i_specify=off  i_priority=None  i=0 A  i_nominal_specify=off  i_nominal_unit=A  i_nominal_value=1  v_specify=off  v_priority=None  v=0 V  v_nominal_specify=off  v_nominal_unit=V  v_nominal_value=1
      settings: AttributesFormatString=|
      | %<dc_voltage>%<dc_voltage_unit>+
      | %<ac_voltage>%<ac_voltage_unit>@
      | %<ac_frequency>%<ac_frequency_unit>
  VSrc{1,3,6..7,10..12,15..16,18,21} (11 alike) : nesl_utility/PS-Simulink Converter  PhysicalDomain=network_engine_domain  SubClassName=ps_output  LeftPortType=input  RightPortType=output  PseudoPeriodic=off  Frequencies=[]  VectorFormat=1-D array  Unit=V  AffineConversion=off
  VSrc{2,4..5,8..9,13..14,17,19..20,22} (11 alike) : nesl_utility/PS-Simulink Converter  PhysicalDomain=network_engine_domain  SubClassName=ps_output  LeftPortType=input  RightPortType=output  PseudoPeriodic=off  Frequencies=[]  VectorFormat=1-D array  Unit=A  AffineConversion=off
  Vh10rms_d : Display
  Vh10rms_s : Scope
  Vh1rms_d : Display
  Vh1rms_s : Scope
  Vh2rms_d : Display
  Vh2rms_s : Scope
  Vh3rms_d : Display
  Vh3rms_s : Scope
  Vh4rms_d : Display
  Vh4rms_s : Scope
  Vh5rms_d : Display
  Vh5rms_s : Scope
  Vh6rms_d : Display
  Vh6rms_s : Scope
  Vh7rms_d : Display
  Vh7rms_s : Scope
  Vh8rms_d : Display
  Vh8rms_s : Scope
  Vh9rms_d : Display
  Vh9rms_s : Scope
  Voltage Sensor{,1..10} (11 alike) : fl_lib/Electrical/Electrical Sensors/Voltage Sensor
  Voltage Display {1..30} (30 alike) : Display
  Vtr : Scope
  wires:
  VSrc1/1 -> RMS21/1, Vtr/1
  VSrc12/1 -> RMS4/1
  RMS4/1 -> Complex to Real-Imag1/1, Vh1rms_d/1, Vh1rms_s/1
  RMS1/1 -> Complex to Real-Imag3/1, Ih1rms_s2/1, Ih1rms_d/1
  Complex to Real-Imag3/1 -> Power Measurement1/1
  Complex to Real-Imag1/1 -> Power Measurement1/2
  Power Measurement1/1 -> Ph1rms_s/1, Ph1rms_d/1
  VSrc13/1 -> RMS22/1, Itr/1, Ih1rms_d3/1
  VSrc2/1 -> Ih1rms_s1/1, RMS1/1
  RMS2/1 -> Ih2rms_s2/1, Ih2rms_d/1, Complex to Real-Imag4/1
  VSrc14/1 -> Ih2rms_s1/1, RMS2/1
  Power Measurement2/1 -> Ph2rms_s/1, Ph2rms_d/1
  RMS3/1 -> Complex to Real-Imag2/1, Vh2rms_d/1, Vh2rms_s/1
  Complex to Real-Imag2/1 -> Power Measurement2/2
  Complex to Real-Imag4/1 -> Power Measurement2/1
  VSrc3/1 -> RMS3/1
  RMS6/1 -> Complex to Real-Imag5/1, Vh3rms_d/1, Vh3rms_s/1
  Power Measurement3/1 -> Ph3rms_s/1, Ph3rms_d/1
  VSrc15/1 -> RMS6/1
  RMS5/1 -> Complex to Real-Imag6/1, Ih3rms_s2/1, Ih3rms_d/1
  VSrc4/1 -> Ih3rms_s1/1, RMS5/1
  Complex to Real-Imag6/1 -> Power Measurement3/1
  Complex to Real-Imag5/1 -> Power Measurement3/2
  Power Measurement4/1 -> Ph4rms_s/1, Ph4rms_d/1
  VSrc16/1 -> RMS8/1
  RMS7/1 -> Ih4rms_s2/1, Ih4rms_d/1, Complex to Real-Imag8/1
  Complex to Real-Imag8/1 -> Power Measurement4/1
  Complex to Real-Imag7/1 -> Power Measurement4/2
  VSrc5/1 -> Ih4rms_s1/1, RMS7/1
  RMS8/1 -> Complex to Real-Imag7/1, Vh4rms_d/1, Vh4rms_s/1
  VSrc6/1 -> RMS9/1
  Power Measurement5/1 -> Ph5rms_d/1, Ph5rms_s/1
  RMS10/1 -> Complex to Real-Imag10/1, Ih5rms_s2/1, Ih5rms_d/1
  Complex to Real-Imag10/1 -> Power Measurement5/1
  Complex to Real-Imag9/1 -> Power Measurement5/2
  VSrc17/1 -> RMS10/1, Ih5rms_s1/1
  RMS9/1 -> Vh5rms_s/1, Complex to Real-Imag9/1, Vh5rms_d/1
  VSrc7/1 -> RMS11/1
  RMS12/1 -> Complex to Real-Imag11/1, Ih6rms_s2/1, Ih6rms_d/1
  Power Measurement6/1 -> Ph6rms_d/1, Ph6rms_s/1
  VSrc8/1 -> RMS12/1, Ih6rms_s1/1
  Complex to Real-Imag12/1 -> Power Measurement6/2
  Complex to Real-Imag11/1 -> Power Measurement6/1
  RMS11/1 -> Vh6rms_s/1, Complex to Real-Imag12/1, Vh6rms_d/1
  VSrc18/1 -> RMS13/1
  Complex to Real-Imag14/1 -> Power Measurement7/2
  Complex to Real-Imag13/1 -> Power Measurement7/1
  VSrc19/1 -> RMS14/1, Ih7rms_s1/1
  RMS14/1 -> Complex to Real-Imag13/1, Ih7rms_s2/1, Ih7rms_d/1
  RMS13/1 -> Vh7rms_s/1, Complex to Real-Imag14/1, Vh7rms_d/1
  Power Measurement7/1 -> Ph7rms_d/1, Ph7rms_s/1
  RMS15/1 -> Complex to Real-Imag15/1, Ih8rms_s2/1, Ih8rms_d/1
  RMS16/1 -> Complex to Real-Imag16/1, Vh8rms_d/1, Vh8rms_s/1
  Power Measurement8/1 -> Ph8rms_d/1, Ph8rms_s/1
  VSrc20/1 -> RMS15/1, Ih8rms_s1/1
  VSrc21/1 -> RMS16/1
  Complex to Real-Imag16/1 -> Power Measurement8/2
  Complex to Real-Imag15/1 -> Power Measurement8/1
  Power Measurement9/1 -> Ph9rms_d/1, Ph9rms_s/1
  RMS18/1 -> Complex to Real-Imag18/1, Vh9rms_d/1, Vh9rms_s/1
  VSrc10/1 -> RMS18/1
  RMS17/1 -> Complex to Real-Imag17/1, Ih9rms_s2/1, Ih9rms_d/1
  VSrc9/1 -> RMS17/1, Ih9rms_s1/1
  Complex to Real-Imag17/1 -> Power Measurement9/1
  Complex to Real-Imag18/1 -> Power Measurement9/2
  Complex to Real-Imag20/1 -> Power Measurement10/2
  Complex to Real-Imag19/1 -> Power Measurement10/1
  VSrc11/1 -> RMS20/1
  VSrc22/1 -> RMS19/1, Ih10rms_s1/1
  RMS19/1 -> Complex to Real-Imag19/1, Ih10rms_s2/1, Ih10rms_d/1
  RMS20/1 -> Complex to Real-Imag20/1, Vh10rms_d/1, Vh10rms_s/1
  Power Measurement10/1 -> Ph10rms_d/1, Ph10rms_s/1
  From Workspace/1 -> MATLAB Function11/2(ws)
  Constant11/1 -> Divide11/2
  MATLAB Function11/1(y) -> Divide11/1
  Digital Clock11/1 -> MATLAB Function11/1(time)
  Divide11/1 -> Product11/1, Scope5/1, Voltage Display 2/1
  Complex to Real-Imag1/2 -> Ph1rms_s1V/1
  Sine Wave11/1 -> Product11/2
  Product11/1 -> Simulink-PS Converter/1
  Constant1/1 -> Divide1/2
  Product1/1 -> Simulink-PS Converter1/1
  Digital Clock1/1 -> MATLAB Function1/1(time)
  From Workspace1/1 -> MATLAB Function1/2(ws)
  MATLAB Function1/1(y) -> Divide1/1
  Divide1/1 -> Scope1/1, Voltage Display 1/1, Product1/1
  Sine Wave1/1 -> Product1/2
  Product2/1 -> Simulink-PS Converter3/1
  MATLAB Function3/1(y) -> Divide3/1
  Constant2/1 -> Divide2/2
  Sine Wave2/1 -> Product2/2
  Product3/1 -> Simulink-PS Converter2/1
  Divide3/1 -> Scope3/1, Voltage Display 4/1, Product3/1
  Constant3/1 -> Divide3/2
  Sine Wave3/1 -> Product3/2
  Digital Clock3/1 -> MATLAB Function3/1(time)
  Digital Clock2/1 -> MATLAB Function2/1(time)
  From Workspace2/1 -> MATLAB Function3/2(ws)
  Divide2/1 -> Scope2/1, Voltage Display 3/1, Product2/1
  From Workspace3/1 -> MATLAB Function2/2(ws)
  MATLAB Function2/1(y) -> Divide2/1
  Product5/1 -> Simulink-PS Converter4/1
  Divide5/1 -> Scope6/1, Voltage Display 6/1, Product5/1
  Product4/1 -> Simulink-PS Converter5/1
  Sine Wave5/1 -> Product5/2
  Sine Wave4/1 -> Product4/2
  Constant4/1 -> Divide4/2
  From Workspace4/1 -> MATLAB Function5/2(ws)
  Constant5/1 -> Divide5/2
  Digital Clock4/1 -> MATLAB Function4/1(time)
  Divide4/1 -> Scope4/1, Voltage Display 5/1, Product4/1
  From Workspace5/1 -> MATLAB Function4/2(ws)
  Digital Clock5/1 -> MATLAB Function5/1(time)
  MATLAB Function5/1(y) -> Divide5/1
  MATLAB Function4/1(y) -> Divide4/1
  From Workspace7/1 -> MATLAB Function6/2(ws)
  Divide6/1 -> Scope7/1, Voltage Display 7/1, Product6/1
  Constant7/1 -> Divide7/2
  MATLAB Function6/1(y) -> Divide6/1
  MATLAB Function7/1(y) -> Divide7/1
  From Workspace6/1 -> MATLAB Function7/2(ws)
  Digital Clock6/1 -> MATLAB Function6/1(time)
  Divide7/1 -> Scope8/1, Voltage Display 8/1, Product7/1
  Digital Clock7/1 -> MATLAB Function7/1(time)
  Product7/1 -> Simulink-PS Converter6/1
  Product6/1 -> Simulink-PS Converter7/1
  Constant6/1 -> Divide6/2
  Sine Wave7/1 -> Product7/2
  Sine Wave6/1 -> Product6/2
  Constant13/1 -> Divide13/2
  Digital Clock15/1 -> MATLAB Function15/1(time)
  Constant15/1 -> Divide15/2
  Sine Wave15/1 -> Product15/2
  Sine Wave16/1 -> Product16/2
  Sine Wave14/1 -> Product14/2
  Divide13/1 -> Scope12/1, Voltage Display 13/1, Product13/1
  Product16/1 -> Simulink-PS Converter14/1
  From Workspace15/1 -> MATLAB Function15/2(ws)
  Digital Clock12/1 -> MATLAB Function12/1(time)
  Sine Wave10/1 -> Product10/2
  Product12/1 -> Simulink-PS Converter10/1
  Digital Clock16/1 -> MATLAB Function16/1(time)
  From Workspace9/1 -> MATLAB Function8/2(ws)
  Divide16/1 -> Scope16/1, Voltage Display 16/1, Product16/1
  Constant16/1 -> Divide16/2
  From Workspace13/1 -> MATLAB Function13/2(ws)
  MATLAB Function16/1(y) -> Divide16/1
  From Workspace12/1 -> MATLAB Function14/2(ws)
  From Workspace14/1 -> MATLAB Function16/2(ws)
  Divide14/1 -> Scope14/1, Voltage Display 14/1, Product14/1
  MATLAB Function15/1(y) -> Divide15/1
  Digital Clock13/1 -> MATLAB Function13/1(time)
  MATLAB Function14/1(y) -> Divide14/1
  Product13/1 -> Simulink-PS Converter13/1
  Digital Clock10/1 -> MATLAB Function10/1(time)
  Constant14/1 -> Divide14/2
  MATLAB Function10/1(y) -> Divide10/1
  Divide10/1 -> Scope10/1, Voltage Display 11/1, Product10/1
  From Workspace10/1 -> MATLAB Function12/2(ws)
  Sine Wave12/1 -> Product12/2
  Constant10/1 -> Divide10/2
  MATLAB Function12/1(y) -> Divide12/1
  Product15/1 -> Simulink-PS Converter15/1
  Sine Wave8/1 -> Product8/2
  Product10/1 -> Simulink-PS Converter11/1
  Divide8/1 -> Scope9/1, Voltage Display 9/1, Product8/1
  Divide15/1 -> Scope15/1, Voltage Display 15/1, Product15/1
  Digital Clock8/1 -> MATLAB Function8/1(time)
  Sine Wave13/1 -> Product13/2
  Product8/1 -> Simulink-PS Converter9/1
  Constant8/1 -> Divide8/2
  Product14/1 -> Simulink-PS Converter12/1
  MATLAB Function8/1(y) -> Divide8/1
  Digital Clock9/1 -> MATLAB Function9/1(time)
  Constant12/1 -> Divide12/2
  Product9/1 -> Simulink-PS Converter8/1
  MATLAB Function9/1(y) -> Divide9/1
  Sine Wave9/1 -> Product9/2
  MATLAB Function13/1(y) -> Divide13/1
  From Workspace8/1 -> MATLAB Function9/2(ws)
  Divide12/1 -> Scope11/1, Voltage Display 12/1, Product12/1
  Constant9/1 -> Divide9/2
  From Workspace11/1 -> MATLAB Function10/2(ws)
  Digital Clock14/1 -> MATLAB Function14/1(time)
  Divide9/1 -> Scope13/1, Voltage Display 10/1, Product9/1
  Product17/1 -> Simulink-PS Converter17/1
  MATLAB Function17/1(y) -> Divide17/1
  Constant18/1 -> Divide18/2
  From Workspace16/1 -> MATLAB Function18/2(ws)
  MATLAB Function18/1(y) -> Divide18/1
  Digital Clock18/1 -> MATLAB Function18/1(time)
  Divide18/1 -> Scope18/1, Product18/1, Voltage Display 18/1
  Divide17/1 -> Scope17/1, Product17/1, Voltage Display 17/1
  Sine Wave18/1 -> Product18/2
  From Workspace17/1 -> MATLAB Function17/2(ws)
  Constant17/1 -> Divide17/2
  Sine Wave17/1 -> Product17/2
  Product18/1 -> Simulink-PS Converter16/1
  Digital Clock17/1 -> MATLAB Function17/1(time)
  MATLAB Function19/1(y) -> Divide19/1
  Constant20/1 -> Divide20/2
  From Workspace18/1 -> MATLAB Function20/2(ws)
  MATLAB Function20/1(y) -> Divide20/1
  Digital Clock20/1 -> MATLAB Function20/1(time)
  Divide20/1 -> Scope20/1, Product20/1, Voltage Display 20/1
  Divide19/1 -> Scope19/1, Product19/1, Voltage Display 19/1
  Sine Wave20/1 -> Product20/2
  From Workspace19/1 -> MATLAB Function19/2(ws)
  Constant19/1 -> Divide19/2
  Sine Wave19/1 -> Product19/2
  Product20/1 -> Simulink-PS Converter18/1
  Digital Clock19/1 -> MATLAB Function19/1(time)
  Complex to Real-Imag10/2 -> Ph5rms_s5I/1
  Complex to Real-Imag9/2 -> Ph5rms_s5V/1
  Complex to Real-Imag12/2 -> Ph6rms_s6V/1
  Complex to Real-Imag11/2 -> Ph6rms_s6I/1
  Complex to Real-Imag14/2 -> Ph7rms_s7V/1
  Complex to Real-Imag13/2 -> Ph7rms_s7I/1
  Complex to Real-Imag20/2 -> Ph10rms_s10V/1
  Complex to Real-Imag19/2 -> Ph10rms_s10I/1
  Complex to Real-Imag18/2 -> Ph9rms_s9V/1
  Complex to Real-Imag17/2 -> Ph9rms_s9I/1
  Complex to Real-Imag16/2 -> Ph8rms_s8V/1
  Complex to Real-Imag15/2 -> Ph8rms_s8I/1
  Complex to Real-Imag2/2 -> Ph2rms_s2V/1
  Complex to Real-Imag4/2 -> Ph2rms_s2I/1
  Complex to Real-Imag3/2 -> Ph1rms_s1I/1
  Complex to Real-Imag6/2 -> Ph3rms_s3I/1
  Complex to Real-Imag5/2 -> Ph3rms_s3V/1
  Complex to Real-Imag8/2 -> Ph4rms_s4I/1
  Complex to Real-Imag7/2 -> Ph4rms_s4V/1
  Power Measurement1/2 -> Ph1rms_s1/1
  Power Measurement2/2 -> Ph2rms_s2/1
  Power Measurement3/2 -> Ph3rms_s3/1
  Power Measurement4/2 -> Ph4rms_s4/1
  Power Measurement5/2 -> Ph5rms_s5/1
  Power Measurement6/2 -> Ph6rms_s6/1
  Power Measurement7/2 -> Ph1rms_s7/1
  Power Measurement8/2 -> Ph8rms_s8/1
  Power Measurement9/2 -> Ph9rms_s9/1
  Power Measurement10/2 -> Ph10rms_s10/1
  From Workspace20/1 -> MATLAB Function21/2(ws)
  Constant21/1 -> Divide21/2
  MATLAB Function21/1(y) -> Divide21/1
  Divide21/1 -> Scope21/1, Voltage Display 21/1, Product21/1
  Digital Clock21/1 -> MATLAB Function21/1(time)
  Sine Wave21/1 -> Product21/2
  From Workspace21/1 -> MATLAB Function22/2(ws)
  Constant22/1 -> Divide22/2
  MATLAB Function22/1(y) -> Divide22/1
  Divide22/1 -> Scope22/1, Voltage Display 22/1, Product22/1
  Digital Clock22/1 -> MATLAB Function22/1(time)
  Sine Wave22/1 -> Product22/2
  Product22/1 -> Simulink-PS Converter21/1
  From Workspace22/1 -> MATLAB Function23/2(ws)
  Constant23/1 -> Divide23/2
  MATLAB Function23/1(y) -> Divide23/1
  Divide23/1 -> Scope23/1, Voltage Display 23/1, Product23/1
  Digital Clock23/1 -> MATLAB Function23/1(time)
  Sine Wave23/1 -> Product23/2
  Product23/1 -> Simulink-PS Converter22/1
  From Workspace23/1 -> MATLAB Function24/2(ws)
  Constant24/1 -> Divide24/2
  MATLAB Function24/1(y) -> Divide24/1
  Divide24/1 -> Scope24/1, Voltage Display 24/1, Product24/1
  Digital Clock24/1 -> MATLAB Function24/1(time)
  Sine Wave24/1 -> Product24/2
  Product24/1 -> Simulink-PS Converter23/1
  From Workspace24/1 -> MATLAB Function25/2(ws)
  Constant25/1 -> Divide25/2
  MATLAB Function25/1(y) -> Divide25/1
  Divide25/1 -> Scope25/1, Product25/1, Voltage Display 25/1
  Digital Clock25/1 -> MATLAB Function25/1(time)
  Sine Wave25/1 -> Product25/2
  From Workspace25/1 -> MATLAB Function26/2(ws)
  Constant26/1 -> Divide26/2
  MATLAB Function26/1(y) -> Divide26/1
  Divide26/1 -> Scope26/1, Product26/1, Voltage Display 26/1
  Digital Clock26/1 -> MATLAB Function26/1(time)
  Sine Wave26/1 -> Product26/2
  From Workspace26/1 -> MATLAB Function27/2(ws)
  Constant27/1 -> Divide27/2
  MATLAB Function27/1(y) -> Divide27/1
  Divide27/1 -> Scope27/1, Product27/1, Voltage Display 27/1
  Digital Clock27/1 -> MATLAB Function27/1(time)
  Sine Wave27/1 -> Product27/2
  From Workspace27/1 -> MATLAB Function28/2(ws)
  Constant28/1 -> Divide28/2
  MATLAB Function28/1(y) -> Divide28/1
  Divide28/1 -> Scope28/1, Voltage Display 28/1, Product28/1
  Digital Clock28/1 -> MATLAB Function28/1(time)
  Sine Wave28/1 -> Product28/2
  Product28/1 -> Simulink-PS Converter24/1
  From Workspace28/1 -> MATLAB Function29/2(ws)
  Constant29/1 -> Divide29/2
  MATLAB Function29/1(y) -> Divide29/1
  Divide29/1 -> Scope29/1, Voltage Display 29/1, Product29/1
  Digital Clock29/1 -> MATLAB Function29/1(time)
  Sine Wave29/1 -> Product29/2
  Product29/1 -> Simulink-PS Converter25/1
  From Workspace29/1 -> MATLAB Function30/2(ws)
  Constant30/1 -> Divide30/2
  MATLAB Function30/1(y) -> Divide30/1
  Divide30/1 -> Scope30/1, Voltage Display 30/1, Product30/1
  Digital Clock30/1 -> MATLAB Function30/1(time)
  Sine Wave30/1 -> Product30/2
  Product30/1 -> Simulink-PS Converter26/1
  Product21/1 -> Simulink-PS Converter20/1
  Product25/1 -> Simulink-PS Converter27/1
  Product26/1 -> Simulink-PS Converter28/1
  Product27/1 -> Simulink-PS Converter29/1
  Constant31/1 -> Product11/3
  Product19/1 -> Simulink-PS Converter19/1
  Constant32/1 -> Product1/3
  Constant33/1 -> Product21/3
  Constant34/1 -> Product22/3
  Constant35/1 -> Product2/3
  Constant36/1 -> Product3/3
  Constant37/1 -> Product5/3
  Constant38/1 -> Product4/3
  Constant39/1 -> Product23/3
  Constant40/1 -> Product24/3
  Constant41/1 -> Product6/3
  Constant42/1 -> Product7/3
  Constant43/1 -> Product15/3
  Constant44/1 -> Product16/3
  Constant45/1 -> Product25/3
  Constant46/1 -> Product17/3
  Constant47/1 -> Product18/3
  Constant48/1 -> Product26/3
  Constant49/1 -> Product19/3
  Constant50/1 -> Product20/3
  Constant51/1 -> Product27/3
  Constant52/1 -> Product30/3
  Constant53/1 -> Product14/3
  Constant54/1 -> Product13/3
  Constant55/1 -> Product29/3
  Constant56/1 -> Product12/3
  Constant57/1 -> Product10/3
  Constant58/1 -> Product28/3
  Constant59/1 -> Product9/3
  Constant60/1 -> Product8/3
  Complex to Real-Imag21/1 -> Power Measurement11/2
  Complex to Real-Imag22/1 -> Power Measurement11/1
  Power Measurement11/1 -> Ph1rms_s2/1, Ph1rms_d1/1
  RMS22/1 -> Itr1/1, Complex to Real-Imag21/1, Ih1rms_d2/1
  RMS21/1 -> Complex to Real-Imag22/1, Ih1rms_s3/1, Ih1rms_d1/1
  connections:
  Current Sensor10/RConn2 -- -Line Pair 9 (AMKA 35 85 m)/LConn1 -- Line Pair 1 (AMKA 35 89 m)/LConn1
  Inductor/LConn1 -- Line Pair 1 (AMKA 35 89 m)/RConn1
  Inductor1/LConn1 -- Line Pair House 1 (MC 10 38 m)/RConn1
  Inductor1/RConn1 -- Voltage Sensor1/LConn1 -- PV_1/LConn1 -- EV_1/RConn2 -- Controlled Current Source/RConn2
  Controlled Current Source/LConn1 -- EV_1/LConn1 -- PV_1/RConn2 -- Current Sensor/LConn1
  VSrc2/LConn1 -- Current Sensor/RConn1
  Inductor2/LConn1 -- Line Pair 2 (AMKA 35 60 m)/RConn1
  Inductor3/LConn1 -- Line Pair 3 (AMKA 35 95 m)/RConn1
  -Line Pair House 3(MC 10 34 m)/LConn1 -- Line Pair 4 (AXMK 50 571 m)/LConn1 -- Inductor3/RConn1
  Inductor2/RConn1 -- Line Pair 3 (AMKA 35 95 m)/LConn1 -- -Line Pair House 2(MC 10 48 m)/LConn1
  Inductor5/LConn1 -- -Line Pair House 2(MC 10 48 m)/RConn1
  PV_2/RConn2 -- Controlled Current Source1/LConn1 -- Current Sensor1/LConn1 -- EV_2/LConn1
  EV_2/RConn2 -- Voltage Sensor2/LConn1 -- Inductor5/RConn1 -- Controlled Current Source1/RConn2 -- PV_2/LConn1
  Inductor6/LConn1 -- -Line Pair House 3(MC 10 34 m)/RConn1
  PV_3/RConn2 -- Current Sensor2/LConn1 -- Controlled Current Source2/LConn1 -- EV_3/LConn1
  EV_3/RConn2 -- Controlled Current Source2/RConn2 -- Inductor6/RConn1 -- Voltage Sensor3/LConn1 -- PV_3/LConn1
  -Line Pair House 4(MC6  4 m)/LConn1 -- Inductor4/RConn1
  Inductor7/LConn1 -- -Line Pair House 4(MC6  4 m)/RConn1
  EV_4/RConn2 -- Controlled Current Source3/RConn2 -- Inductor7/RConn1 -- Voltage Sensor4/LConn1 -- PV_4/LConn1
  Inductor4/LConn1 -- Line Pair 4 (AXMK 50 571 m)/RConn1
  Line Pair 8 (AMKA 35 33 m)/LConn1 -- Line Pair 6 (AMKA 16 45 m)/LConn1 -- Line Pair 7 (AMKA 35 137 m)/LConn1 -- Inductor9/RConn1
  Inductor9/LConn1 -- Line Pair 5 (AMKA 35 248 m)/RConn1
  Inductor12/LConn1 -- Line Pair 8 (AMKA 35 33 m)/RConn1
  Inductor10/LConn1 -- Line Pair 6 (AMKA 16 45 m)/RConn1
  Inductor11/LConn1 -- Line Pair 7 (AMKA 35 137 m)/RConn1
  Inductor13/LConn1 -- -Line Pair House 5(MC 6 11 m)/RConn1
  EV_5/RConn2 -- Controlled Current Source4/RConn2 -- Inductor13/RConn1 -- Voltage Sensor5/LConn1 -- PV_5/LConn1
  -Line Pair House 5(MC 6 11 m)/LConn1 -- Inductor10/RConn1
  Inductor14/LConn1 -- -Line Pair House 6(MC 10 12 m)/RConn1
  EV_6/RConn2 -- Controlled Current Source5/RConn2 -- Voltage Sensor6/LConn1 -- Inductor14/RConn1 -- PV_6/LConn1
  -Line Pair House 6(MC 10 12 m)/LConn1 -- Inductor11/RConn1
  EV_7/RConn2 -- Controlled Current Source6/RConn2 -- Inductor15/RConn1 -- Voltage Sensor7/LConn1 -- PV_7/LConn1
  Inductor12/RConn1 -- Line Pair House 7(MC 10 38 m)/LConn1
  Inductor15/LConn1 -- Line Pair House 7(MC 10 38 m)/RConn1
  -Line Pair 9 (AMKA 35 85 m)/RConn1 -- Inductor8/LConn1
  Inductor16/RConn1 -- Voltage Sensor8/LConn1 -- EV_8/RConn2 -- PV_8/LConn1 -- Controlled Current Source7/RConn2
  Inductor16/LConn1 -- Line Pair House 8 (MC 10 29 m)/RConn1
  Controlled Current Source7/LConn1 -- EV_8/LConn1 -- PV_8/RConn2 -- Current Sensor7/LConn1
  Line Pair House 8 (MC 10 29 m)/LConn1 -- -Line Pair 10 (AMKA 35 52 m)/LConn1 -- Inductor8/RConn1
  -Line Pair 10 (AMKA 35 52 m)/RConn1 -- Inductor17/LConn1
  Inductor18/LConn1 -- Line Pair House 9 (MC 10 35 m)/RConn1
  Inductor17/RConn1 -- -Line Pair 11 (AMKA 25 58 m)/LConn1 -- Line Pair House 9 (MC 10 35 m)/LConn1
  -Line Pair 11 (AMKA 25 58 m)/RConn1 -- Inductor19/LConn1
  PV_10/LConn1 -- Voltage Sensor10/LConn1 -- Inductor20/RConn1 -- Controlled Current Source9/RConn2 -- EV_10/RConn2
  Inductor20/LConn1 -- Line Pair House 10 (MC 6 40 m)/RConn1
  Inductor19/RConn1 -- Line Pair House 10 (MC 6 40 m)/LConn1
  VSrc/LConn1 -- Voltage Sensor/LConn1 -- Current Sensor10/LConn1
  VSrc13/LConn1 -- Current Sensor10/RConn1
  Inductor/RConn1 -- Line Pair 2 (AMKA 35 60 m)/LConn1 -- Line Pair 5 (AMKA 35 248 m)/LConn1 -- Line Pair House 1 (MC 10 38 m)/LConn1
  VSrc1/LConn1 -- Voltage Sensor/RConn1
  Voltage Sensor1/RConn1 -- VSrc12/LConn1
  Voltage Sensor2/RConn1 -- VSrc3/LConn1
  VSrc14/LConn1 -- Current Sensor1/RConn1
  VSrc4/LConn1 -- Current Sensor2/RConn1
  Voltage Sensor3/RConn1 -- VSrc15/LConn1
  PV_4/RConn2 -- Controlled Current Source3/LConn1 -- Current Sensor3/LConn1 -- EV_4/LConn1
  Current Sensor3/RConn1 -- VSrc5/LConn1
  Voltage Sensor4/RConn1 -- VSrc16/LConn1
  EV_5/LConn1 -- PV_5/RConn2 -- Controlled Current Source4/LConn1 -- Current Sensor4/LConn1
  Voltage Sensor5/RConn1 -- VSrc6/LConn1
  VSrc17/LConn1 -- Current Sensor4/RConn1
  Voltage Sensor7/RConn2 -- Current Sensor6/RConn2 -- Current Sensor5/RConn2 -- Voltage Sensor6/RConn2 -- Current Sensor4/RConn2 -- Voltage Sensor5/RConn2 -- Current Sensor3/RConn2 -- Voltage Sensor4/RConn2 -- Voltage Sensor8/RConn2 -- Voltage Sensor9/RConn2 -- Voltage Sensor10/RConn2 -- Current Sensor9/RConn2 -- Current Sensor8/RConn2 -- Current Sensor7/RConn2 -- Solver Configuration/RConn1 -- VSrc/RConn1 -- ERef/LConn1 -- Voltage Sensor/RConn2 -- Voltage Sensor1/RConn2 -- Current Sensor/RConn2 -- Voltage Sensor2/RConn2 -- Current Sensor1/RConn2 -- Voltage Sensor3/RConn2 -- Current Sensor2/RConn2
  Voltage Sensor6/RConn1 -- VSrc7/LConn1
  VSrc8/LConn1 -- Current Sensor5/RConn1
  PV_6/RConn2 -- Current Sensor5/LConn1 -- Controlled Current Source5/LConn1 -- EV_6/LConn1
  PV_7/RConn2 -- Current Sensor6/LConn1 -- Controlled Current Source6/LConn1 -- EV_7/LConn1
  Voltage Sensor7/RConn1 -- VSrc18/LConn1
  VSrc19/LConn1 -- Current Sensor6/RConn1
  Voltage Sensor8/RConn1 -- VSrc21/LConn1
  VSrc20/LConn1 -- Current Sensor7/RConn1
  PV_9/LConn1 -- Controlled Current Source8/RConn2 -- Voltage Sensor9/LConn1 -- Inductor18/RConn1 -- EV_9/RConn2
  PV_9/RConn2 -- Current Sensor8/LConn1 -- Controlled Current Source8/LConn1 -- EV_9/LConn1
  Voltage Sensor9/RConn1 -- VSrc10/LConn1
  Current Sensor8/RConn1 -- VSrc9/LConn1
  PV_10/RConn2 -- Current Sensor9/LConn1 -- Controlled Current Source9/LConn1 -- EV_10/LConn1
  Current Sensor9/RConn1 -- VSrc22/LConn1
  Voltage Sensor10/RConn1 -- VSrc11/LConn1
  Controlled Current Source/RConn1 -- Simulink-PS Converter/RConn1
  Simulink-PS Converter2/RConn1 -- Controlled Current Source1/RConn1
  Simulink-PS Converter3/RConn1 -- PV_2/RConn1
  Simulink-PS Converter4/RConn1 -- Controlled Current Source2/RConn1
  Simulink-PS Converter5/RConn1 -- PV_3/RConn1
  Simulink-PS Converter6/RConn1 -- Controlled Current Source3/RConn1
  Simulink-PS Converter7/RConn1 -- PV_4/RConn1
  PV_5/RConn1 -- Simulink-PS Converter15/RConn1
  Simulink-PS Converter14/RConn1 -- Controlled Current Source4/RConn1
  Simulink-PS Converter17/RConn1 -- PV_6/RConn1
  Simulink-PS Converter16/RConn1 -- Controlled Current Source5/RConn1
  Simulink-PS Converter18/RConn1 -- Controlled Current Source6/RConn1
  Simulink-PS Converter9/RConn1 -- PV_8/RConn1
  Simulink-PS Converter8/RConn1 -- Controlled Current Source7/RConn1
  Simulink-PS Converter11/RConn1 -- PV_9/RConn1
  Simulink-PS Converter10/RConn1 -- Controlled Current Source8/RConn1
  Simulink-PS Converter13/RConn1 -- PV_10/RConn1
  Simulink-PS Converter12/RConn1 -- Controlled Current Source9/RConn1
  PV_1/RConn1 -- Simulink-PS Converter1/RConn1
  Simulink-PS Converter20/RConn1 -- EV_1/RConn1
  Simulink-PS Converter21/RConn1 -- EV_2/RConn1
  Simulink-PS Converter22/RConn1 -- EV_3/RConn1
  Simulink-PS Converter23/RConn1 -- EV_4/RConn1
  Simulink-PS Converter24/RConn1 -- EV_8/RConn1
  Simulink-PS Converter25/RConn1 -- EV_9/RConn1
  Simulink-PS Converter26/RConn1 -- EV_10/RConn1
  Simulink-PS Converter27/RConn1 -- EV_5/RConn1
  EV_6/RConn1 -- Simulink-PS Converter28/RConn1
  Simulink-PS Converter29/RConn1 -- EV_7/RConn1
  Simulink-PS Converter19/RConn1 -- PV_7/RConn1
